simulink model "tdc_model_01"  (R2018a)
settings: Solver=VariableStepAuto  StartTime=0.0  StopTime=30.0  RelTol=1e-3
settings Model: Creator=Nicolas  LastModifiedBy=Nicolas

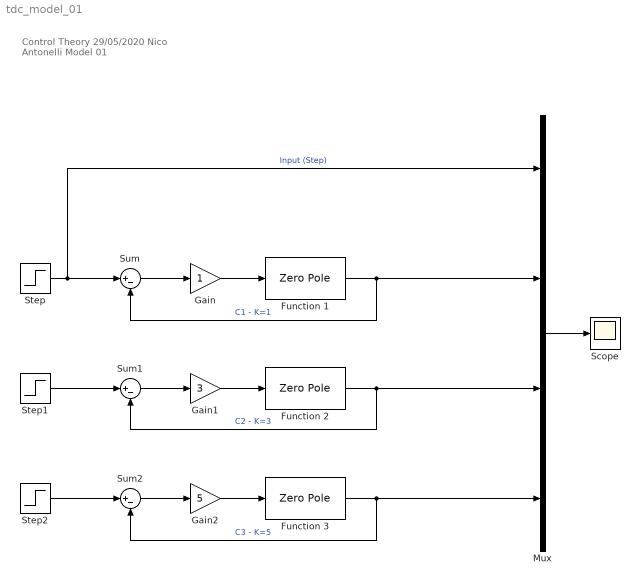
== system tdc_model_01 ==
  note: Control Theory
      | 29/05/2020
      | Nico Antonelli
      |
      | Model 01
  Function 1 : ZeroPole  Zeros=[]  Poles=[-1 -1 -1]
  Function 2 : ZeroPole  Zeros=[]  Poles=[-1 -1 -1]
  Function 3 : ZeroPole  Zeros=[]  Poles=[-1 -1 -1]
  Gain : Gain
  Gain1 : Gain  Gain=3
  Gain2 : Gain  Gain=5
  Mux : Mux
  Scope : Scope
  Step : Step  SampleTime=0
  Step1 : Step  SampleTime=0
  Step2 : Step  SampleTime=0
  Sum : Sum  Inputs=|+-
  Sum1 : Sum  Inputs=|+-
  Sum2 : Sum  Inputs=|+-
  wires:
  Step/1 -> Mux/1, Sum/1  "Input (Step)"
  Sum/1 -> Gain/1
  Gain/1 -> Function 1/1
  Function 1/1 -> Sum/2, Mux/2  "C1 - K=1"
  Mux/1 -> Scope/1
  Step1/1 -> Sum1/1
  Function 2/1 -> Sum1/2, Mux/3  "C2 - K=3"
  Gain1/1 -> Function 2/1
  Sum1/1 -> Gain1/1
  Sum2/1 -> Gain2/1
  Gain2/1 -> Function 3/1
  Function 3/1 -> Mux/4, Sum2/2  "C3 - K=5"
  Step2/1 -> Sum2/1
